simulink model "k1visetmxp"  (Simulink 8.6)
settings: Solver=ode45  StartTime=0.0  StopTime=10.0  RelTol=1e-3
libraries: cdsIPCx x51, cdsFilt x7, cdsCDI64 x6, cdsCDO64 x6, BIO_CD_DECODE_MASTER x6, BIO_CD_ENCODE_MASTER x5, CHK_DIO x5, dac x3, VIS_LIB x3, cdsBit2Word x2, cdsAdcx0 x1, cdsAdcx1 x1
settings Model: Creator=controls  LastModifiedBy=controls
settings DataIOCC: SignalLoggingSaveFormat=Dataset
settings OptimizationCC: ExpressionDepthLimit=128
settings DebuggingCC: UnderspecifiedInitializationDetection=Simplified  MergeDetectMultiDrivingBlocksExec=error  SolverPrmCheckMsg=none  FcnCallInpInsideContextMsg=EnableAllAsError  StateNameClashWarn=none
settings GRTTargetCC: CombineOutputUpdateFcns=on  GRTInterface=off

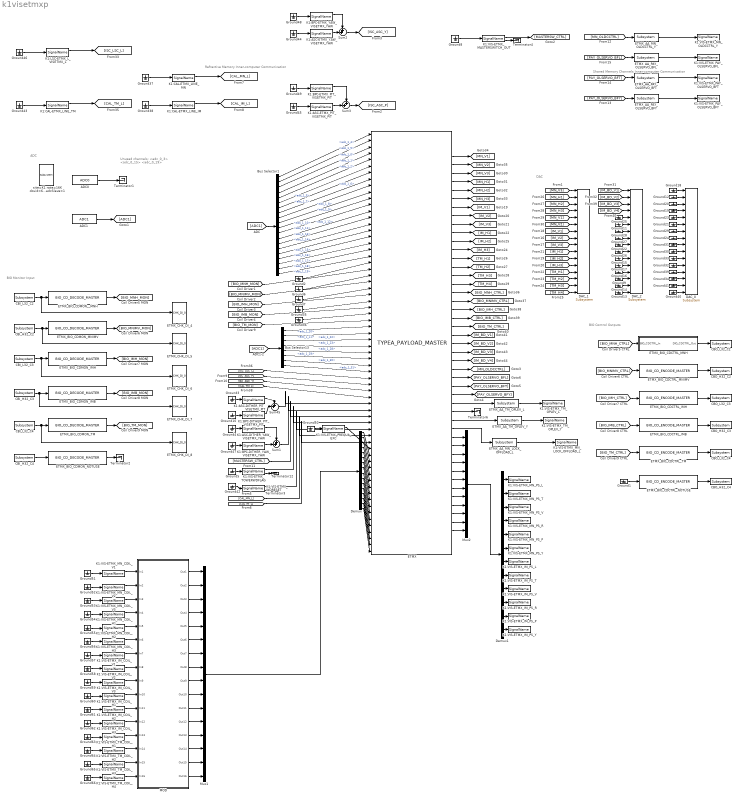
== system k1visetmxp ==
  note: BIO Monitor Input
  note: BIO Control Outputs
  note: DAC
  note: ADC
  note: Refrective Memory
      | Inner-computer Communication
  note: Unused channels:
      | <adc_0_3>
      | <adc_0_15>
      | <adc_0_19>
  note: Shared Memory Channels
      | Inner-computer Communication
  ADC0 : cdsAdcx0/ADC0  Tag=cdsAdc  Description=|
      | type-GSC_16AI64SSA
      | card_num=0
      settings: AttributesFormatString=%<Description>\n%<Tag>
  ADC1 : cdsAdcx1/ADC1  Tag=cdsAdc  Description=|
      | type-GSC_16AI64SSA
      | card_num=1
      settings: AttributesFormatString=%<Description>\n%<Tag>
  Bus Selector1 : BusSelector  OutputSignals=adc_1_4,adc_1_5,adc_1_0,adc_1_1,adc_1_2,adc_1_3,adc_1_6,adc_1_7,adc_1_8,adc_1_9,adc_1_10,adc_1_11,adc_1_12,adc_1_13,adc_1_14,adc_1_15,adc_1_16,adc_1_17,adc_1_18,adc_1_19
  Bus Selector13 : BusSelector  OutputSignals=adc_1_20,adc_1_21,adc_1_22,adc_1_23,adc_1_28,adc_1_29,adc_1_30,adc_1_31
  CBI_H32_C2 : cdsCDI64/Subsystem  Tag=cdsCDI64  Description=card_num=5
      settings: AttributesFormatString=%<Tag>\n%<Description>
  CBI_H32_C3 : cdsCDI64/Subsystem  Tag=cdsCDI64  Description=card_num=7
      settings: AttributesFormatString=%<Tag>\n%<Description>
  CBI_H32_C4 : cdsCDI64/Subsystem  Tag=cdsCDI64  Description=card_num=9
      settings: AttributesFormatString=%<Tag>\n%<Description>
  CBI_L32_C2 : cdsCDI64/Subsystem  Tag=cdsCDI64  Description=card_num=4
      settings: AttributesFormatString=%<Tag>\n%<Description>
  CBI_L32_C3 : cdsCDI64/Subsystem  Tag=cdsCDI64  Description=card_num=6
      settings: AttributesFormatString=%<Tag>\n%<Description>
  CBI_L32_C4 : cdsCDI64/Subsystem  Tag=cdsCDI64  Description=card_num=8
      settings: AttributesFormatString=%<Tag>\n%<Description>
  CBO_H32_C2 : cdsCDO64/Subsystem  Tag=cdsCDO64  Description=card_num=5
      settings: AttributesFormatString=%<Tag>\n%<Description>
  CBO_H32_C3 : cdsCDO64/Subsystem  Tag=cdsCDO64  Description=card_num=7
      settings: AttributesFormatString=%<Tag>\n%<Description>
  CBO_H32_C4 : cdsCDO64/Subsystem  Tag=cdsCDO64  Description=card_num=9
      settings: AttributesFormatString=%<Tag>\n%<Description>
  CBO_L32_C2 : cdsCDO64/Subsystem  Tag=cdsCDO64  Description=card_num=4
      settings: AttributesFormatString=%<Tag>\n%<Description>
  CBO_L32_C3 : cdsCDO64/Subsystem  Tag=cdsCDO64  Description=card_num=6
      settings: AttributesFormatString=%<Tag>\n%<Description>
  CBO_L32_C4 : cdsCDO64/Subsystem  Tag=cdsCDO64  Description=card_num=8
      settings: AttributesFormatString=%<Tag>\n%<Description>
  DAC_0 : dac/Subsystem  Description=|
      | type=GSC_16AO16,
      | card_num=0
      settings: AttributesFormatString=%<Description>
  DAC_1 : dac/Subsystem  Description=|
      | type=GSC_16AO16,
      | card_num=1
      settings: AttributesFormatString=%<Description>
  DAC_2 : dac/Subsystem  Description=|
      | type=GSC_16AO16,
      | card_num=2
      settings: AttributesFormatString=%<Description>
  Demux : Demux  Outputs=16
  Demux1 : Demux  Outputs=12
  ETMX : TYPEA_MASTER/TYPEA_PAYLOAD_MASTER
  ETMX_AA_MN_LOCK_OFFLOAD_L : cdsFilt/Subsystem  Tag=cdsFilt  Description=|
      | Purpose:                                                                                                                                                                                                                                  
      | Standard CDS IIR filter module.                                                                                                                                                                                                           
      |                                                                                                                                                                                                                                           
      | Operation:                                                                                                                                                                                                                                
      | Consists of 10 second order section IIR filters, plus a ramped gain stage. In FE code, also provides pre-defined test points and excitation channel inputs. The filter coefficients are defined in the LIGO system using the 'foton' tool.
      |                                                                                                                                                                                                                                           
      | Usage:                                                                                                                                                                                                                                    
      | Name the part with the desired filter module name.
      settings: AttributesFormatString=%<Tag>
  ETMX_AA_MN_OLDCCTRL_Y : cdsFilt/Subsystem  Tag=cdsFilt  Description=|
      | Purpose:                                                                                                                                                                                                                                  
      | Standard CDS IIR filter module.                                                                                                                                                                                                           
      |                                                                                                                                                                                                                                           
      | Operation:                                                                                                                                                                                                                                
      | Consists of 10 second order section IIR filters, plus a ramped gain stage. In FE code, also provides pre-defined test points and excitation channel inputs. The filter coefficients are defined in the LIGO system using the 'foton' tool.
      |                                                                                                                                                                                                                                           
      | Usage:                                                                                                                                                                                                                                    
      | Name the part with the desired filter module name.
      settings: AttributesFormatString=%<Tag>
  ETMX_AA_PAY_OLSERVO_BFL : cdsFilt/Subsystem  Tag=cdsFilt  Description=|
      | Purpose:                                                                                                                                                                                                                                  
      | Standard CDS IIR filter module.                                                                                                                                                                                                           
      |                                                                                                                                                                                                                                           
      | Operation:                                                                                                                                                                                                                                
      | Consists of 10 second order section IIR filters, plus a ramped gain stage. In FE code, also provides pre-defined test points and excitation channel inputs. The filter coefficients are defined in the LIGO system using the 'foton' tool.
      |                                                                                                                                                                                                                                           
      | Usage:                                                                                                                                                                                                                                    
      | Name the part with the desired filter module name.
      settings: AttributesFormatString=%<Tag>
  ETMX_AA_PAY_OLSERVO_BFT : cdsFilt/Subsystem  Tag=cdsFilt  Description=|
      | Purpose:                                                                                                                                                                                                                                  
      | Standard CDS IIR filter module.                                                                                                                                                                                                           
      |                                                                                                                                                                                                                                           
      | Operation:                                                                                                                                                                                                                                
      | Consists of 10 second order section IIR filters, plus a ramped gain stage. In FE code, also provides pre-defined test points and excitation channel inputs. The filter coefficients are defined in the LIGO system using the 'foton' tool.
      |                                                                                                                                                                                                                                           
      | Usage:                                                                                                                                                                                                                                    
      | Name the part with the desired filter module name.
      settings: AttributesFormatString=%<Tag>
  ETMX_AA_PAY_OLSERVO_BFY : cdsFilt/Subsystem  Tag=cdsFilt  Description=|
      | Purpose:                                                                                                                                                                                                                                  
      | Standard CDS IIR filter module.                                                                                                                                                                                                           
      |                                                                                                                                                                                                                                           
      | Operation:                                                                                                                                                                                                                                
      | Consists of 10 second order section IIR filters, plus a ramped gain stage. In FE code, also provides pre-defined test points and excitation channel inputs. The filter coefficients are defined in the LIGO system using the 'foton' tool.
      |                                                                                                                                                                                                                                           
      | Usage:                                                                                                                                                                                                                                    
      | Name the part with the desired filter module name.
      settings: AttributesFormatString=%<Tag>
  ETMX_AA_TM_OPLEV_L : cdsFilt/Subsystem  Tag=cdsFilt  Description=|
      | Purpose:                                                                                                                                                                                                                                  
      | Standard CDS IIR filter module.                                                                                                                                                                                                           
      |                                                                                                                                                                                                                                           
      | Operation:                                                                                                                                                                                                                                
      | Consists of 10 second order section IIR filters, plus a ramped gain stage. In FE code, also provides pre-defined test points and excitation channel inputs. The filter coefficients are defined in the LIGO system using the 'foton' tool.
      |                                                                                                                                                                                                                                           
      | Usage:                                                                                                                                                                                                                                    
      | Name the part with the desired filter module name.
      settings: AttributesFormatString=%<Tag>
  ETMX_AA_TM_OPLEV_Y : cdsFilt/Subsystem  Tag=cdsFilt  Description=|
      | Purpose:                                                                                                                                                                                                                                  
      | Standard CDS IIR filter module.                                                                                                                                                                                                           
      |                                                                                                                                                                                                                                           
      | Operation:                                                                                                                                                                                                                                
      | Consists of 10 second order section IIR filters, plus a ramped gain stage. In FE code, also provides pre-defined test points and excitation channel inputs. The filter coefficients are defined in the LIGO system using the 'foton' tool.
      |                                                                                                                                                                                                                                           
      | Usage:                                                                                                                                                                                                                                    
      | Name the part with the desired filter module name.
      settings: AttributesFormatString=%<Tag>
  ETMX_BIO_CDCTRL_IMB : BIO_CD_ENCODE_MASTER/BIO_CD_ENCODE_MASTER
  ETMX_BIO_CDCTRL_IMH : BIO_CD_ENCODE_MASTER/BIO_CD_ENCODE_MASTER
  ETMX_BIO_CDCTRL_MNH : Subsystem
  ETMX_BIO_CDCTRL_MNIMV : BIO_CD_ENCODE_MASTER/BIO_CD_ENCODE_MASTER
  ETMX_BIO_CDCTRL_NOTUSE : BIO_CD_ENCODE_MASTER/BIO_CD_ENCODE_MASTER
  ETMX_BIO_CDCTRL_TM : BIO_CD_ENCODE_MASTER/BIO_CD_ENCODE_MASTER
  ETMX_BIO_CDMON_IMB : BIO_CD_DECODE_MASTER/BIO_CD_DECODE_MASTER
  ETMX_BIO_CDMON_IMH : BIO_CD_DECODE_MASTER/BIO_CD_DECODE_MASTER
  ETMX_BIO_CDMON_MNIMV : BIO_CD_DECODE_MASTER/BIO_CD_DECODE_MASTER
  ETMX_BIO_CDMON_NOTUSE : BIO_CD_DECODE_MASTER/BIO_CD_DECODE_MASTER
  ETMX_BIO_CDMON_TM : BIO_CD_DECODE_MASTER/BIO_CD_DECODE_MASTER
  ETMX_BIO_CDMON__MNH : BIO_CD_DECODE_MASTER/BIO_CD_DECODE_MASTER
  ETMX_CHK_DI_{4..8} (5 alike) : CHK_DIO/CHK_DI_0
  Ground{1..66} (66 alike) : Ground
  K1:ASC-DITHER_PIT_VISETMX_PIT : cdsIPCx/SignalName  Tag=cdsIPCx_RFM  Description=card=0
      settings: AttributesFormatString=%<Description>\n%<Tag>
  K1:ASC-DITHER_YAW_VISETMX_YAW : cdsIPCx/SignalName  Tag=cdsIPCx_RFM  Description=card=0
      settings: AttributesFormatString=%<Description>\n%<Tag>
  K1:ASC-ETMX_PIT_VISETMX_PIT : cdsIPCx/SignalName  Tag=cdsIPCx_RFM  Description=card=0
      settings: AttributesFormatString=%<Description>\n%<Tag>
  K1:ASC-ETMX_YAW_VISETMX_YAW : cdsIPCx/SignalName  Tag=cdsIPCx_RFM  Description=card=0
      settings: AttributesFormatString=%<Description>\n%<Tag>
  K1:BPC-DITHER_PIT_VISETMX_PIT : cdsIPCx/SignalName  Tag=cdsIPCx_RFM  Description=card=0
      settings: AttributesFormatString=%<Description>\n%<Tag>
  K1:BPC-DITHER_YAW_VISETMX_YAW : cdsIPCx/SignalName  Tag=cdsIPCx_RFM  Description=card=0
      settings: AttributesFormatString=%<Description>\n%<Tag>
  K1:BPC-ETMX_PIT_VISETMX_PIT : cdsIPCx/SignalName  Tag=cdsIPCx_RFM  Description=card=0
      settings: AttributesFormatString=%<Description>\n%<Tag>
  K1:BPC-ETMX_YAW_VISETMX_YAW : cdsIPCx/SignalName  Tag=cdsIPCx_RFM  Description=card=0
      settings: AttributesFormatString=%<Description>\n%<Tag>
  K1:CAL-ETMX_LINE_IM : cdsIPCx/SignalName  Tag=cdsIPCx_RFM  Description=card=0
      settings: AttributesFormatString=%<Description>\n%<Tag>
  K1:CAL-ETMX_LINE_MN : cdsIPCx/SignalName  Tag=cdsIPCx_RFM  Description=card=0
      settings: AttributesFormatString=%<Description>\n%<Tag>
  K1:CAL-ETMX_LINE_TM : cdsIPCx/SignalName  Tag=cdsIPCx_RFM  Description=card=0
      settings: AttributesFormatString=%<Description>\n%<Tag>
  K1:LSC-ETMX_L_VISETMX_L : cdsIPCx/SignalName  Tag=cdsIPCx_RFM  Description=card=0
      settings: AttributesFormatString=%<Description>\n%<Tag>
  K1:VIS-ETMX_MASTERSWITCH_OUT : cdsIPCx/SignalName  Tag=cdsIPCx_SHMEM  Description=Inter-Process Communication via Shared memory.
      settings: AttributesFormatString=%<Tag>
  K1:VIS-ETMX_MN_LOCK_OFFLOAD_L : cdsIPCx/SignalName  Tag=cdsIPCx_SHMEM  Description=Inter-Process Communication via Shared memory.
      settings: AttributesFormatString=%<Tag>
  K1:VIS-ETMX_MN_OLDCCTRL_Y : cdsIPCx/SignalName  Tag=cdsIPCx_SHMEM  Description=Inter-Process Communication via Shared memory.
      settings: AttributesFormatString=%<Tag>
  K1:VIS-ETMX_PAY_OLSERVO_BFL : cdsIPCx/SignalName  Tag=cdsIPCx_SHMEM  Description=Inter-Process Communication via Shared memory.
      settings: AttributesFormatString=%<Tag>
  K1:VIS-ETMX_PAY_OLSERVO_BFT : cdsIPCx/SignalName  Tag=cdsIPCx_SHMEM  Description=Inter-Process Communication via Shared memory.
      settings: AttributesFormatString=%<Tag>
  K1:VIS-ETMX_PAY_OLSERVO_BFY : cdsIPCx/SignalName  Tag=cdsIPCx_SHMEM  Description=Inter-Process Communication via Shared memory.
      settings: AttributesFormatString=%<Tag>
  K1:VIS-ETMX_TM_OPLEV_L : cdsIPCx/SignalName  Tag=cdsIPCx_SHMEM  Description=Inter-Process Communication via Shared memory.
      settings: AttributesFormatString=%<Tag>
  K1:VIS-ETMX_TM_OPLEV_Y : cdsIPCx/SignalName  Tag=cdsIPCx_SHMEM  Description=Inter-Process Communication via Shared memory.
      settings: AttributesFormatString=%<Tag>
  K1:VIS-ETMX_TOWERWDFLAG : cdsIPCx/SignalName  Tag=cdsIPCx_SHMEM  Description=Inter-Process Communication via Shared memory.
      settings: AttributesFormatString=%<Tag>
  K1:VIS-ETMX_WDRESET : cdsIPCx/SignalName  Tag=cdsIPCx_SHMEM  Description=Inter-Process Communication via Shared memory.
      settings: AttributesFormatString=%<Tag>
  K1:VIS-ETMX_IM_COIL_H1 : cdsIPCx/SignalName  Tag=cdsIPCx_SHMEM  Description=Inter-Process Communication via Shared memory.
      settings: AttributesFormatString=%<Tag>
  K1:VIS-ETMX_IM_COIL_H2 : cdsIPCx/SignalName  Tag=cdsIPCx_SHMEM  Description=Inter-Process Communication via Shared memory.
      settings: AttributesFormatString=%<Tag>
  K1:VIS-ETMX_IM_COIL_H3 : cdsIPCx/SignalName  Tag=cdsIPCx_SHMEM  Description=Inter-Process Communication via Shared memory.
      settings: AttributesFormatString=%<Tag>
  K1:VIS-ETMX_IM_COIL_V1 : cdsIPCx/SignalName  Tag=cdsIPCx_SHMEM  Description=Inter-Process Communication via Shared memory.
      settings: AttributesFormatString=%<Tag>
  K1:VIS-ETMX_IM_COIL_V2 : cdsIPCx/SignalName  Tag=cdsIPCx_SHMEM  Description=Inter-Process Communication via Shared memory.
      settings: AttributesFormatString=%<Tag>
  K1:VIS-ETMX_IM_COIL_V3 : cdsIPCx/SignalName  Tag=cdsIPCx_SHMEM  Description=Inter-Process Communication via Shared memory.
      settings: AttributesFormatString=%<Tag>
  K1:VIS-ETMX_IM_PS_L : cdsIPCx/SignalName  Tag=cdsIPCx_SHMEM  Description=Inter-Process Communication via Shared memory.
      settings: AttributesFormatString=%<Tag>
  K1:VIS-ETMX_IM_PS_P : cdsIPCx/SignalName  Tag=cdsIPCx_SHMEM  Description=Inter-Process Communication via Shared memory.
      settings: AttributesFormatString=%<Tag>
  K1:VIS-ETMX_IM_PS_R : cdsIPCx/SignalName  Tag=cdsIPCx_SHMEM  Description=Inter-Process Communication via Shared memory.
      settings: AttributesFormatString=%<Tag>
  K1:VIS-ETMX_IM_PS_T : cdsIPCx/SignalName  Tag=cdsIPCx_SHMEM  Description=Inter-Process Communication via Shared memory.
      settings: AttributesFormatString=%<Tag>
  K1:VIS-ETMX_IM_PS_V : cdsIPCx/SignalName  Tag=cdsIPCx_SHMEM  Description=Inter-Process Communication via Shared memory.
      settings: AttributesFormatString=%<Tag>
  K1:VIS-ETMX_IM_PS_Y : cdsIPCx/SignalName  Tag=cdsIPCx_SHMEM  Description=Inter-Process Communication via Shared memory.
      settings: AttributesFormatString=%<Tag>
  K1:VIS-ETMX_MN_COIL_H1 : cdsIPCx/SignalName  Tag=cdsIPCx_SHMEM  Description=Inter-Process Communication via Shared memory.
      settings: AttributesFormatString=%<Tag>
  K1:VIS-ETMX_MN_COIL_H2 : cdsIPCx/SignalName  Tag=cdsIPCx_SHMEM  Description=Inter-Process Communication via Shared memory.
      settings: AttributesFormatString=%<Tag>
  K1:VIS-ETMX_MN_COIL_H3 : cdsIPCx/SignalName  Tag=cdsIPCx_SHMEM  Description=Inter-Process Communication via Shared memory.
      settings: AttributesFormatString=%<Tag>
  K1:VIS-ETMX_MN_COIL_V1 : cdsIPCx/SignalName  Tag=cdsIPCx_SHMEM  Description=Inter-Process Communication via Shared memory.
      settings: AttributesFormatString=%<Tag>
  K1:VIS-ETMX_MN_COIL_V2 : cdsIPCx/SignalName  Tag=cdsIPCx_SHMEM  Description=Inter-Process Communication via Shared memory.
      settings: AttributesFormatString=%<Tag>
  K1:VIS-ETMX_MN_COIL_V3 : cdsIPCx/SignalName  Tag=cdsIPCx_SHMEM  Description=Inter-Process Communication via Shared memory.
      settings: AttributesFormatString=%<Tag>
  K1:VIS-ETMX_MN_PS_L : cdsIPCx/SignalName  Tag=cdsIPCx_SHMEM  Description=Inter-Process Communication via Shared memory.
      settings: AttributesFormatString=%<Tag>
  K1:VIS-ETMX_MN_PS_P : cdsIPCx/SignalName  Tag=cdsIPCx_SHMEM  Description=Inter-Process Communication via Shared memory.
      settings: AttributesFormatString=%<Tag>
  K1:VIS-ETMX_MN_PS_R : cdsIPCx/SignalName  Tag=cdsIPCx_SHMEM  Description=Inter-Process Communication via Shared memory.
      settings: AttributesFormatString=%<Tag>
  K1:VIS-ETMX_MN_PS_T : cdsIPCx/SignalName  Tag=cdsIPCx_SHMEM  Description=Inter-Process Communication via Shared memory.
      settings: AttributesFormatString=%<Tag>
  K1:VIS-ETMX_MN_PS_V : cdsIPCx/SignalName  Tag=cdsIPCx_SHMEM  Description=Inter-Process Communication via Shared memory.
      settings: AttributesFormatString=%<Tag>
  K1:VIS-ETMX_MN_PS_Y : cdsIPCx/SignalName  Tag=cdsIPCx_SHMEM  Description=Inter-Process Communication via Shared memory.
      settings: AttributesFormatString=%<Tag>
  K1:VIS-ETMX_PREQUA_EXC : cdsIPCx/SignalName  Tag=cdsIPCx_SHMEM  Description=Inter-Process Communication via Shared memory.
      settings: AttributesFormatString=%<Tag>
  K1:VIS-ETMX_TM_COIL_H{1..4} (4 alike) : cdsIPCx/SignalName  Tag=cdsIPCx_SHMEM  Description=Inter-Process Communication via Shared memory.
      settings: AttributesFormatString=%<Tag>
  MOD : Subsystem  Tag=top_names
  Mux1 : Mux  Inputs=16
  Mux2 : Mux  Inputs=12
  Sum{1..3,45} (4 alike) : Sum  Inputs=++|
  Terminator{1..4,6,12} (6 alike) : Terminator
  site=K1 rate=16K dcuid=69 host=k1ex1 specific_cpu=3 adcSlave=1 : cdsParameters/Subsystem  Tag=cdsParameters  Description=|
      | Purpose:                                                                                                                                                                                                                                
      | Provide system parameters to the FE code generator to properly configure the generated EPICS names, rep rate of the FE controller, and the Data Acquisition node ID for proper storage of data from this FE controller.                 
      |                                                                                                                                                                                                                                         
      | Useage:                                                                                                                                                                                                                                 
      | The part NAME field is used to identify the FE parameters. It must be of the form:                                                                                                                                                      
      | site=                                                                                                                                                                                                                                   
      | rate=                                                                                                                                                                                                                                   
      | dcuid=                                                                                                                                                                                                                                  
      |                                                                                                                                                                                                                                         
      | Where:                                                                                                                                                                                                                                  
      | site= argument may be H1, H2, L1, M1, G1, either as a single argument or multiple, for example site=H1,H2. These are the only names allowed. These will become the first two characters of all EPICS and signal names (for example G1:).
      |                                                                                                                                                                                                                                         
      | rate= may be 2K, 16K, 32K, or 64K                                                                                                                                                                                                       
      |                                                                                                                                                                                                                                         
      | dcuid= is site specific ie it must be unique at each site.
      settings: AttributesFormatString=%<Tag>
  wires:
  ADC1/1 -> [ADC1]
  ETMX/1 -> [MN_V1]
  ETMX/2 -> [MN_V2]
  ETMX/3 -> [MN_V3]
  ETMX/4 -> [MN_H1]
  ETMX/6 -> [MN_H3]
  ETMX/7 -> [IM_V1]
  ETMX/8 -> [IM_V2]
  ETMX/9 -> [IM_V3]
  ETMX/11 -> [IM_H2]
  ETMX/12 -> [IM_H3]
  ETMX/13 -> [TM_H1]
  ETMX/14 -> [TM_H2]
  ETMX/16 -> [TM_H4]
  ETMX/17 -> [BIO_MNH_CTRL]
  ETMX/19 -> [BIO_IMH_CTRL]
  ETMX/18 -> [BIO_MNIMV_CTRL]
  ETMX/20 -> [BIO_IMB_CTRL]
  ETMX/21 -> [BIO_TM_CTRL]
  [ADC1] -> Bus Selector13/1
  [MN_V3] -> DAC_1/1
  [MN_H1] -> DAC_1/2
  [MN_H2] -> DAC_1/3
  [MN_H3] -> DAC_1/4
  [MN_V1] -> DAC_1/5
  [MN_V2] -> DAC_1/6
  [IM_V1] -> DAC_1/7
  [IM_V2] -> DAC_1/8
  [IM_V3] -> DAC_1/9
  [IM_H1] -> DAC_1/10
  [TM_H1] -> DAC_1/13
  [TM_H4] -> DAC_1/16
  [TM_H3] -> DAC_1/15
  [TM_H2] -> DAC_1/14
  [IM_H2] -> DAC_1/11
  [IM_H3] -> DAC_1/12
  [BIO_MNH_CTRL] -> ETMX_BIO_CDCTRL_MNH/1(BIO_CDCTRL_In)
  ETMX_BIO_CDCTRL_MNH/1(DIO_CDCTRL_Out) -> CBO_L32_C2/1
  [BIO_MNIMV_CTRL] -> ETMX_BIO_CDCTRL_MNIMV/1
  ETMX_BIO_CDCTRL_MNIMV/1 -> CBO_H32_C2/1
  [BIO_IMH_CTRL] -> ETMX_BIO_CDCTRL_IMH/1
  ETMX_BIO_CDCTRL_IMH/1 -> CBO_L32_C3/1
  [BIO_IMB_CTRL] -> ETMX_BIO_CDCTRL_IMB/1
  ETMX_BIO_CDCTRL_IMB/1 -> CBO_H32_C3/1
  [BIO_TM_CTRL] -> ETMX_BIO_CDCTRL_TM/1
  ETMX_BIO_CDCTRL_TM/1 -> CBO_L32_C4/1
  Ground1/1 -> ETMX_BIO_CDCTRL_NOTUSE/1
  ETMX_BIO_CDCTRL_NOTUSE/1 -> CBO_H32_C4/1
  CBI_L32_C2/1 -> ETMX_CHK_DI_4/1, ETMX_BIO_CDMON__MNH/1
  ETMX_BIO_CDMON__MNH/1 -> [BIO_MNH_MON]
  CBI_H32_C2/1 -> ETMX_CHK_DI_5/1, ETMX_BIO_CDMON_MNIMV/1
  ETMX_BIO_CDMON_MNIMV/1 -> [BIO_MNIMV_MON]
  CBI_L32_C3/1 -> ETMX_CHK_DI_6/1, ETMX_BIO_CDMON_IMH/1
  ETMX_BIO_CDMON_IMH/1 -> [BIO_IMH_MON]
  ETMX_BIO_CDMON_IMB/1 -> [BIO_IMB_MON]
  CBI_L32_C4/1 -> ETMX_CHK_DI_8/1, ETMX_BIO_CDMON_TM/1
  ETMX_BIO_CDMON_TM/1 -> [BIO_TM_MON]
  CBI_H32_C4/1 -> ETMX_BIO_CDMON_NOTUSE/1
  ETMX_BIO_CDMON_NOTUSE/1 -> Terminator2/1
  [IM_BD_V1] -> DAC_2/1
  [IM_BD_V2] -> DAC_2/2
  [IM_BD_V3] -> DAC_2/3
  [IM_BD_V4] -> DAC_2/4
  Ground25/1 -> DAC_2/5
  Ground11/1 -> DAC_2/6
  Ground28/1 -> DAC_2/7
  Ground27/1 -> DAC_2/8
  Ground22/1 -> DAC_2/9
  Ground26/1 -> DAC_2/10
  Ground15/1 -> DAC_2/11
  Ground17/1 -> DAC_2/12
  Ground16/1 -> DAC_2/13
  Ground9/1 -> DAC_2/14
  Ground14/1 -> DAC_2/15
  Ground13/1 -> DAC_2/16
  ETMX/22 -> [IM_BD_V1]
  ETMX/23 -> [IM_BD_V2]
  ETMX/24 -> [IM_BD_V3]
  ETMX/25 -> [IM_BD_V4]
  CBI_H32_C3/1 -> ETMX_CHK_DI_7/1, ETMX_BIO_CDMON_IMB/1
  ETMX/5 -> [MN_H2]
  ETMX/10 -> [IM_H1]
  ETMX/15 -> [TM_H3]
  [ADC1] -> Bus Selector1/1
  K1:VIS-ETMX_TOWERWDFLAG/2 -> Terminator12/1
  Ground5/1 -> K1:VIS-ETMX_TOWERWDFLAG/1
  ADC0/1 -> Terminator1/1
  Ground18/1 -> DAC_0/1
  Ground12/1 -> DAC_0/2
  Ground19/1 -> DAC_0/4
  Ground20/1 -> DAC_0/3
  Ground29/1 -> DAC_0/7
  Ground23/1 -> DAC_0/5
  Ground21/1 -> DAC_0/6
  Ground24/1 -> DAC_0/8
  Ground31/1 -> DAC_0/9
  Ground30/1 -> DAC_0/10
  Ground33/1 -> DAC_0/11
  Ground32/1 -> DAC_0/12
  Ground39/1 -> DAC_0/13
  Ground34/1 -> DAC_0/14
  Ground41/1 -> DAC_0/15
  Ground40/1 -> DAC_0/16
  K1:VIS-ETMX_WDRESET/2 -> Terminator3/1
  Ground42/1 -> K1:VIS-ETMX_WDRESET/1
  Ground46/1 -> K1:LSC-ETMX_L_VISETMX_L/1
  K1:LSC-ETMX_L_VISETMX_L/1 -> [ISC_LSC_L]
  K1:CAL-ETMX_LINE_TM/1 -> [CAL_TM_L]
  Ground43/1 -> K1:CAL-ETMX_LINE_TM/1
  K1:CAL-ETMX_LINE_MN/1 -> [CAL_MN_L]
  Ground37/1 -> K1:CAL-ETMX_LINE_MN/1
  K1:CAL-ETMX_LINE_IM/1 -> [CAL_IM_L]
  Ground38/1 -> K1:CAL-ETMX_LINE_IM/1
  Ground44/1 -> K1:ASC-ETMX_YAW_VISETMX_YAW/1
  Ground45/1 -> K1:ASC-ETMX_PIT_VISETMX_PIT/1
  K1:ASC-ETMX_YAW_VISETMX_YAW/1 -> Sum2/2
  K1:ASC-ETMX_PIT_VISETMX_PIT/1 -> Sum3/2
  Ground3/1 -> K1:ASC-DITHER_PIT_VISETMX_PIT/1
  Ground4/1 -> K1:ASC-DITHER_YAW_VISETMX_YAW/1
  ETMX_AA_MN_OLDCCTRL_Y/1 -> K1:VIS-ETMX_MN_OLDCCTRL_Y/1
  ETMX_AA_PAY_OLSERVO_BFY/1 -> K1:VIS-ETMX_PAY_OLSERVO_BFY/1
  ETMX_AA_PAY_OLSERVO_BFT/1 -> K1:VIS-ETMX_PAY_OLSERVO_BFT/1
  ETMX_AA_PAY_OLSERVO_BFL/1 -> K1:VIS-ETMX_PAY_OLSERVO_BFL/1
  [PAY_OLSERVO_BFY] -> ETMX_AA_PAY_OLSERVO_BFY/1
  [PAY_OLSERVO_BFT] -> ETMX_AA_PAY_OLSERVO_BFT/1
  [PAY_OLSERVO_BFL] -> ETMX_AA_PAY_OLSERVO_BFL/1
  [MN_OLDCCTRL] -> ETMX_AA_MN_OLDCCTRL_Y/1
  ETMX_AA_TM_OPLEV_L/1 -> K1:VIS-ETMX_TM_OPLEV_L/1
  ETMX_AA_TM_OPLEV_Y/1 -> K1:VIS-ETMX_TM_OPLEV_Y/1
  Bus Selector13/1 -> ETMX/31  "<adc_1_20>"
  Bus Selector13/2 -> ETMX/32  "<adc_1_21>"
  Bus Selector13/3 -> ETMX/33  "<adc_1_22>"
  Bus Selector1/19 -> ETMX/19  "<adc_1_18>"
  Bus Selector1/20 -> ETMX/20  "<adc_1_19>"
  Bus Selector1/5 -> ETMX/5  "<adc_1_2>"
  Bus Selector1/16 -> ETMX/16  "<adc_1_15>"
  Bus Selector1/17 -> ETMX/17  "<adc_1_16>"
  Bus Selector1/18 -> ETMX/18  "<adc_1_17>"
  Bus Selector13/4 -> ETMX/34  "<adc_1_23>"
  Bus Selector13/5 -> ETMX/35  "<adc_1_28>"
  Bus Selector13/6 -> ETMX/36  "<adc_1_29>"
  Bus Selector13/7 -> ETMX/37  "<adc_1_30>"
  Bus Selector1/3 -> ETMX/3  "<adc_1_0>"
  Bus Selector1/10 -> ETMX/10  "<adc_1_9>"
  Bus Selector1/11 -> ETMX/11  "<adc_1_10>"
  Bus Selector1/8 -> ETMX/8  "<adc_1_7>"
  Bus Selector1/9 -> ETMX/9  "<adc_1_8>"
  Bus Selector1/14 -> ETMX/14  "<adc_1_13>"
  Bus Selector1/15 -> ETMX/15  "<adc_1_14>"
  Bus Selector1/12 -> ETMX/12  "<adc_1_11>"
  Bus Selector1/13 -> ETMX/13  "<adc_1_12>"
  Bus Selector1/4 -> ETMX/4  "<adc_1_1>"
  Bus Selector1/2 -> ETMX/2  "<adc_1_5>"
  Bus Selector1/1 -> ETMX/1  "<adc_1_4>"
  Bus Selector13/8 -> ETMX/38  "<adc_1_31>"
  Bus Selector1/6 -> ETMX/6  "<adc_1_3>"
  Bus Selector1/7 -> ETMX/7  "<adc_1_6>"
  Ground35/1 -> ETMX/27
  Ground36/1 -> ETMX/29
  Ground2/1 -> ETMX/21
  Ground6/1 -> ETMX/23
  Ground7/1 -> ETMX/25
  [ISC_ASC_Y] -> ETMX/41
  [ISC_ASC_P] -> ETMX/40
  [ISC_LSC_L] -> ETMX/39
  [BIO_IMB_MON] -> ETMX/28
  [BIO_TM_MON] -> ETMX/30
  [BIO_MNH_MON] -> ETMX/22
  [BIO_MNIMV_MON] -> ETMX/24
  [BIO_IMH_MON] -> ETMX/26
  [CAL_IM_L] -> ETMX/49
  ETMX/26 -> [MN_OLDCCTRL]
  ETMX/27 -> [PAY_OLSERVO_BFL]
  ETMX/28 -> [PAY_OLSERVO_BFT]
  ETMX/29 -> [PAY_OLSERVO_BFY]
  ETMX/30 -> ETMX_AA_TM_OPLEV_L/1
  ETMX/31 -> Terminator6/1
  ETMX/32 -> ETMX_AA_TM_OPLEV_Y/1
  K1:VIS-ETMX_MASTERSWITCH_OUT/1 -> [MASTERSW_CTRL]
  Ground8/1 -> K1:VIS-ETMX_MASTERSWITCH_OUT/1
  K1:VIS-ETMX_MASTERSWITCH_OUT/2 -> Terminator4/1
  ETMX_AA_MN_LOCK_OFFLOAD_L/1 -> K1:VIS-ETMX_MN_LOCK_OFFLOAD_L/1
  ETMX/33 -> ETMX_AA_MN_LOCK_OFFLOAD_L/1
  [CAL_TM_L] -> ETMX/42
  K1:ASC-DITHER_PIT_VISETMX_PIT/1 -> Sum45/1
  K1:ASC-DITHER_YAW_VISETMX_YAW/1 -> Sum1/1
  [MASTERSW_CTRL] -> ETMX/45
  K1:VIS-ETMX_TOWERWDFLAG/1 -> ETMX/46
  K1:VIS-ETMX_WDRESET/1 -> ETMX/47
  [CAL_MN_L] -> ETMX/48
  Ground10/1 -> K1:BPC-DITHER_PIT_VISETMX_PIT/1
  Ground47/1 -> K1:BPC-DITHER_YAW_VISETMX_YAW/1
  K1:BPC-DITHER_PIT_VISETMX_PIT/1 -> Sum45/2
  Sum45/1 -> ETMX/43
  K1:BPC-DITHER_YAW_VISETMX_YAW/1 -> Sum1/2
  Sum1/1 -> ETMX/44
  Ground48/1 -> K1:BPC-ETMX_YAW_VISETMX_YAW/1
  Ground49/1 -> K1:BPC-ETMX_PIT_VISETMX_PIT/1
  Sum2/1 -> [ISC_ASC_Y]
  K1:BPC-ETMX_YAW_VISETMX_YAW/1 -> Sum2/1
  Sum3/1 -> [ISC_ASC_P]
  K1:BPC-ETMX_PIT_VISETMX_PIT/1 -> Sum3/1
  Mux1/1 -> Demux/1
  Ground51/1 -> K1:VIS-ETMX_MN_COIL_V1/1
  Ground66/1 -> K1:VIS-ETMX_TM_COIL_H4/1
  Ground52/1 -> K1:VIS-ETMX_MN_COIL_V2/1
  Ground53/1 -> K1:VIS-ETMX_MN_COIL_V3/1
  Ground54/1 -> K1:VIS-ETMX_MN_COIL_H1/1
  Ground55/1 -> K1:VIS-ETMX_MN_COIL_H2/1
  Ground56/1 -> K1:VIS-ETMX_MN_COIL_H3/1
  Ground57/1 -> K1:VIS-ETMX_IM_COIL_V1/1
  Ground58/1 -> K1:VIS-ETMX_IM_COIL_V2/1
  Ground59/1 -> K1:VIS-ETMX_IM_COIL_V3/1
  Ground60/1 -> K1:VIS-ETMX_IM_COIL_H1/1
  Ground61/1 -> K1:VIS-ETMX_IM_COIL_H2/1
  Ground62/1 -> K1:VIS-ETMX_IM_COIL_H3/1
  Ground63/1 -> K1:VIS-ETMX_TM_COIL_H1/1
  Ground64/1 -> K1:VIS-ETMX_TM_COIL_H2/1
  Ground65/1 -> K1:VIS-ETMX_TM_COIL_H3/1
  MOD/1(Out1) -> Mux1/1
  MOD/2(Out2) -> Mux1/2
  MOD/3(Out3) -> Mux1/3
  MOD/4(Out4) -> Mux1/4
  MOD/5(Out5) -> Mux1/5
  MOD/6(Out6) -> Mux1/6
  MOD/7(Out7) -> Mux1/7
  MOD/8(Out8) -> Mux1/8
  MOD/9(Out9) -> Mux1/9
  MOD/10(Out10) -> Mux1/10
  MOD/11(Out11) -> Mux1/11
  MOD/12(Out12) -> Mux1/12
  MOD/13(Out13) -> Mux1/13
  MOD/14(Out14) -> Mux1/14
  MOD/15(Out15) -> Mux1/15
  MOD/16(Out16) -> Mux1/16
  K1:VIS-ETMX_MN_COIL_V1/1 -> MOD/1(In1)
  K1:VIS-ETMX_MN_COIL_V2/1 -> MOD/2(In2)
  K1:VIS-ETMX_MN_COIL_V3/1 -> MOD/3(In3)
  K1:VIS-ETMX_MN_COIL_H1/1 -> MOD/4(In4)
  K1:VIS-ETMX_MN_COIL_H2/1 -> MOD/5(In5)
  K1:VIS-ETMX_MN_COIL_H3/1 -> MOD/6(In6)
  K1:VIS-ETMX_IM_COIL_V1/1 -> MOD/7(In7)
  K1:VIS-ETMX_IM_COIL_V2/1 -> MOD/8(In8)
  K1:VIS-ETMX_IM_COIL_V3/1 -> MOD/9(In9)
  K1:VIS-ETMX_IM_COIL_H1/1 -> MOD/10(In10)
  K1:VIS-ETMX_IM_COIL_H2/1 -> MOD/11(In11)
  K1:VIS-ETMX_IM_COIL_H3/1 -> MOD/12(In12)
  K1:VIS-ETMX_TM_COIL_H1/1 -> MOD/13(In13)
  K1:VIS-ETMX_TM_COIL_H2/1 -> MOD/14(In14)
  K1:VIS-ETMX_TM_COIL_H3/1 -> MOD/15(In15)
  K1:VIS-ETMX_TM_COIL_H4/1 -> MOD/16(In16)
  Demux/1 -> ETMX/51
  Demux/2 -> ETMX/52
  Demux/3 -> ETMX/53
  Demux/4 -> ETMX/54
  Demux/5 -> ETMX/55
  Demux/6 -> ETMX/56
  Demux/7 -> ETMX/57
  Demux/8 -> ETMX/58
  Demux/9 -> ETMX/59
  Demux/10 -> ETMX/60
  Demux/11 -> ETMX/61
  Demux/12 -> ETMX/62
  Demux/13 -> ETMX/63
  Demux/14 -> ETMX/64
  Demux/15 -> ETMX/65
  Demux/16 -> ETMX/66
  Ground50/1 -> K1:VIS-ETMX_PREQUA_EXC/1
  K1:VIS-ETMX_PREQUA_EXC/1 -> ETMX/50
  Demux1/1 -> K1:VIS-ETMX_MN_PS_L/1
  Demux1/2 -> K1:VIS-ETMX_MN_PS_T/1
  Demux1/3 -> K1:VIS-ETMX_MN_PS_V/1
  Demux1/4 -> K1:VIS-ETMX_MN_PS_R/1
  Demux1/5 -> K1:VIS-ETMX_MN_PS_P/1
  Demux1/6 -> K1:VIS-ETMX_MN_PS_Y/1
  Demux1/7 -> K1:VIS-ETMX_IM_PS_L/1
  Demux1/8 -> K1:VIS-ETMX_IM_PS_T/1
  Demux1/9 -> K1:VIS-ETMX_IM_PS_V/1
  Demux1/10 -> K1:VIS-ETMX_IM_PS_R/1
  Demux1/11 -> K1:VIS-ETMX_IM_PS_P/1
  Demux1/12 -> K1:VIS-ETMX_IM_PS_Y/1
  Mux2/1 -> Demux1/1
  ETMX/34 -> Mux2/1
  ETMX/35 -> Mux2/2
  ETMX/36 -> Mux2/3
  ETMX/37 -> Mux2/4
  ETMX/38 -> Mux2/5
  ETMX/39 -> Mux2/6
  ETMX/40 -> Mux2/7
  ETMX/41 -> Mux2/8
  ETMX/42 -> Mux2/9
  ETMX/43 -> Mux2/10
  ETMX/44 -> Mux2/11
  ETMX/45 -> Mux2/12

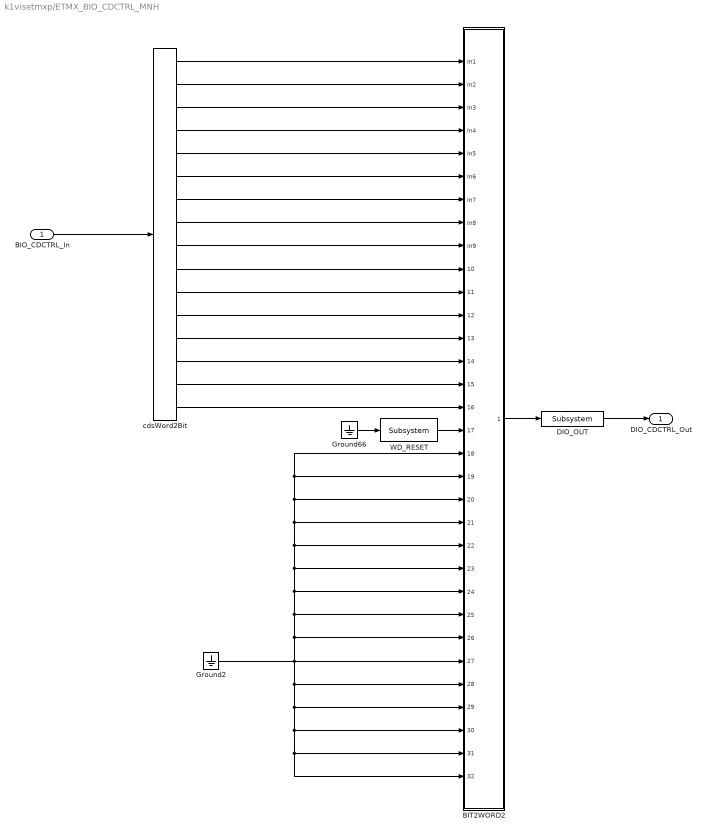
== system k1visetmxp/ETMX_BIO_CDCTRL_MNH ==
  BIO_CDCTRL_In : Inport
  BIT2WORD2 : Subsystem
  DIO_OUT : cdsEpicsOut/Subsystem  Tag=cdsEpicsOutput  Description=|
      | Purpose:                                          
      | Output a FE signal to an EPICS channel.           
      |                                                   
      | Operation:                                        
      | Takes input value and passes it to EPICS record.  
      |                                                   
      | Usage:                                            
      | Name the part with the desired EPICS rrecord name.
      settings: AttributesFormatString=%<Tag>
  Ground2 : Ground
  Ground66 : Ground
  WD_RESET : cdsEpicsBinIn/Subsystem  Tag=cdsEpicsBinIn  Description=|
      | Purpose:                                                                            
      | Create an EPICS binary (0 or 1) input channel to the FE realtime controls.          
      |                                                                                     
      | Operation:                                                                          
      | Outputs value from an EPICS ai record. Value is binary input (bi Epics record type).
      |                                                                                     
      | Usage:                                                                              
      | Name the part with the desired EPICS channel name.
      settings: AttributesFormatString=%<Tag>
  cdsWord2Bit : cdsWord2Bit/cdsWord2Bit  Tag=cdsWord2Bit  Description=Generate 16 0/1 outputs from single 16-bit integer input
      settings: AttributesFormatString=cdsWord2Bit
  DIO_CDCTRL_Out : Outport
  wires:
  BIT2WORD2/1(Out1) -> DIO_OUT/1
  DIO_OUT/1 -> DIO_CDCTRL_Out/1
  BIO_CDCTRL_In/1 -> cdsWord2Bit/1
  cdsWord2Bit/1 -> BIT2WORD2/1(In1)
  cdsWord2Bit/2 -> BIT2WORD2/2(In2)
  cdsWord2Bit/3 -> BIT2WORD2/3(In3)
  cdsWord2Bit/4 -> BIT2WORD2/4(In4)
  cdsWord2Bit/5 -> BIT2WORD2/5(In5)
  cdsWord2Bit/6 -> BIT2WORD2/6(In6)
  cdsWord2Bit/7 -> BIT2WORD2/7(In7)
  cdsWord2Bit/8 -> BIT2WORD2/8(In8)
  cdsWord2Bit/9 -> BIT2WORD2/9(In9)
  cdsWord2Bit/10 -> BIT2WORD2/10(In10)
  cdsWord2Bit/11 -> BIT2WORD2/11(In11)
  cdsWord2Bit/12 -> BIT2WORD2/12(In12)
  cdsWord2Bit/13 -> BIT2WORD2/13(In13)
  cdsWord2Bit/14 -> BIT2WORD2/14(In14)
  cdsWord2Bit/15 -> BIT2WORD2/15(In15)
  cdsWord2Bit/16 -> BIT2WORD2/16(In16)
  WD_RESET/1 -> BIT2WORD2/17(In17)
  Ground66/1 -> WD_RESET/1
  Ground2/1 -> BIT2WORD2/27(In27), BIT2WORD2/28(In28), BIT2WORD2/29(In29), BIT2WORD2/30(In30), BIT2WORD2/31(In31), BIT2WORD2/32(In32), BIT2WORD2/26(In26), BIT2WORD2/25(In25), BIT2WORD2/24(In24), BIT2WORD2/23(In23), BIT2WORD2/22(In22), BIT2WORD2/21(In21), BIT2WORD2/20(In20), BIT2WORD2/18(In18), BIT2WORD2/19(In19)

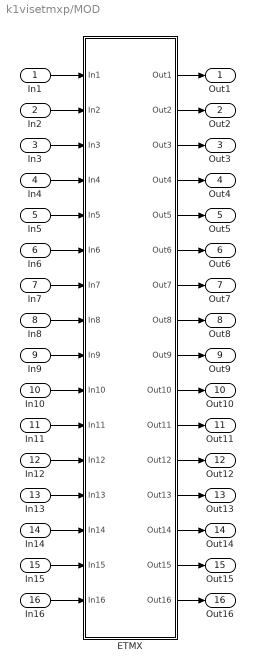
== system k1visetmxp/MOD ==
  In1 : Inport
  In2 : Inport  Port=2
  In3 : Inport  Port=3
  In4 : Inport  Port=4
  In5 : Inport  Port=5
  In6 : Inport  Port=6
  In7 : Inport  Port=7
  In8 : Inport  Port=8
  In9 : Inport  Port=9
  In10 : Inport  Port=10
  In11 : Inport  Port=11
  In12 : Inport  Port=12
  In13 : Inport  Port=13
  In14 : Inport  Port=14
  In15 : Inport  Port=15
  In16 : Inport  Port=16
  ETMX : Subsystem
  Out1 : Outport
  Out2 : Outport  Port=2
  Out3 : Outport  Port=3
  Out4 : Outport  Port=4
  Out5 : Outport  Port=5
  Out6 : Outport  Port=6
  Out7 : Outport  Port=7
  Out8 : Outport  Port=8
  Out9 : Outport  Port=9
  Out10 : Outport  Port=10
  Out11 : Outport  Port=11
  Out12 : Outport  Port=12
  Out13 : Outport  Port=13
  Out14 : Outport  Port=14
  Out15 : Outport  Port=15
  Out16 : Outport  Port=16
  wires:
  In1/1 -> ETMX/1(In1)
  In2/1 -> ETMX/2(In2)
  In3/1 -> ETMX/3(In3)
  In4/1 -> ETMX/4(In4)
  In5/1 -> ETMX/5(In5)
  In6/1 -> ETMX/6(In6)
  In7/1 -> ETMX/7(In7)
  In8/1 -> ETMX/8(In8)
  In9/1 -> ETMX/9(In9)
  In10/1 -> ETMX/10(In10)
  In11/1 -> ETMX/11(In11)
  In12/1 -> ETMX/12(In12)
  In13/1 -> ETMX/13(In13)
  In14/1 -> ETMX/14(In14)
  In15/1 -> ETMX/15(In15)
  In16/1 -> ETMX/16(In16)
  ETMX/1(Out1) -> Out1/1
  ETMX/2(Out2) -> Out2/1
  ETMX/3(Out3) -> Out3/1
  ETMX/4(Out4) -> Out4/1
  ETMX/5(Out5) -> Out5/1
  ETMX/6(Out6) -> Out6/1
  ETMX/7(Out7) -> Out7/1
  ETMX/8(Out8) -> Out8/1
  ETMX/9(Out9) -> Out9/1
  ETMX/10(Out10) -> Out10/1
  ETMX/11(Out11) -> Out11/1
  ETMX/12(Out12) -> Out12/1
  ETMX/13(Out13) -> Out13/1
  ETMX/14(Out14) -> Out14/1
  ETMX/15(Out15) -> Out15/1
  ETMX/16(Out16) -> Out16/1

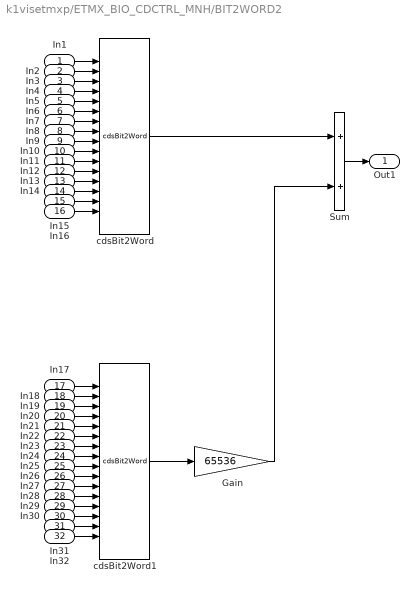
== system k1visetmxp/ETMX_BIO_CDCTRL_MNH/BIT2WORD2 ==
  In1 : Inport
  In2 : Inport  Port=2
  In3 : Inport  Port=3
  In4 : Inport  Port=4
  In5 : Inport  Port=5
  In6 : Inport  Port=6
  In7 : Inport  Port=7
  In8 : Inport  Port=8
  In9 : Inport  Port=9
  In10 : Inport  Port=10
  In11 : Inport  Port=11
  In12 : Inport  Port=12
  In13 : Inport  Port=13
  In14 : Inport  Port=14
  In15 : Inport  Port=15
  In16 : Inport  Port=16
  In17 : Inport  Port=17
  In18 : Inport  Port=18
  In19 : Inport  Port=19
  In20 : Inport  Port=20
  In21 : Inport  Port=21
  In22 : Inport  Port=22
  In23 : Inport  Port=23
  In24 : Inport  Port=24
  In25 : Inport  Port=25
  In26 : Inport  Port=26
  In27 : Inport  Port=27
  In28 : Inport  Port=28
  In29 : Inport  Port=29
  In30 : Inport  Port=30
  In31 : Inport  Port=31
  In32 : Inport  Port=32
  Gain : Gain  Gain=65536
  Sum : Sum
  cdsBit2Word : cdsBit2Word/cdsBit2Word  Tag=cdsBit2Word  Description=Forms single 16 bit integer from 16 0/1 inputs.
      settings: AttributesFormatString=%<Tag>
  cdsBit2Word1 : cdsBit2Word/cdsBit2Word  Tag=cdsBit2Word  Description=Forms single 16 bit integer from 16 0/1 inputs.
      settings: AttributesFormatString=%<Tag>
  Out1 : Outport
  wires:
  In32/1 -> cdsBit2Word1/16
  In31/1 -> cdsBit2Word1/15
  In30/1 -> cdsBit2Word1/14
  In29/1 -> cdsBit2Word1/13
  In28/1 -> cdsBit2Word1/12
  In27/1 -> cdsBit2Word1/11
  In26/1 -> cdsBit2Word1/10
  In25/1 -> cdsBit2Word1/9
  In24/1 -> cdsBit2Word1/8
  In23/1 -> cdsBit2Word1/7
  In22/1 -> cdsBit2Word1/6
  In21/1 -> cdsBit2Word1/5
  In20/1 -> cdsBit2Word1/4
  In19/1 -> cdsBit2Word1/3
  In18/1 -> cdsBit2Word1/2
  In17/1 -> cdsBit2Word1/1
  In16/1 -> cdsBit2Word/16
  In15/1 -> cdsBit2Word/15
  In14/1 -> cdsBit2Word/14
  In13/1 -> cdsBit2Word/13
  In12/1 -> cdsBit2Word/12
  In11/1 -> cdsBit2Word/11
  Sum/1 -> Out1/1
  In10/1 -> cdsBit2Word/10
  In9/1 -> cdsBit2Word/9
  In8/1 -> cdsBit2Word/8
  In7/1 -> cdsBit2Word/7
  In6/1 -> cdsBit2Word/6
  In5/1 -> cdsBit2Word/5
  In4/1 -> cdsBit2Word/4
  In3/1 -> cdsBit2Word/3
  In2/1 -> cdsBit2Word/2
  In1/1 -> cdsBit2Word/1
  cdsBit2Word/1 -> Sum/1
  cdsBit2Word1/1 -> Gain/1
  Gain/1 -> Sum/2

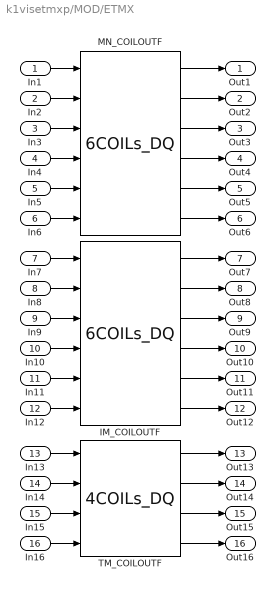
== system k1visetmxp/MOD/ETMX ==
  In1 : Inport
  In2 : Inport  Port=2
  In3 : Inport  Port=3
  In4 : Inport  Port=4
  In5 : Inport  Port=5
  In6 : Inport  Port=6
  In7 : Inport  Port=7
  In8 : Inport  Port=8
  In9 : Inport  Port=9
  In10 : Inport  Port=10
  In11 : Inport  Port=11
  In12 : Inport  Port=12
  In13 : Inport  Port=13
  In14 : Inport  Port=14
  In15 : Inport  Port=15
  In16 : Inport  Port=16
  IM_COILOUTF : VIS_LIB/UTILs/6COILs_DQ
  MN_COILOUTF : VIS_LIB/UTILs/6COILs_DQ
  TM_COILOUTF : VIS_LIB/UTILs/4COILs_DQ
  Out1 : Outport
  Out2 : Outport  Port=2
  Out3 : Outport  Port=3
  Out4 : Outport  Port=4
  Out5 : Outport  Port=5
  Out6 : Outport  Port=6
  Out7 : Outport  Port=7
  Out8 : Outport  Port=8
  Out9 : Outport  Port=9
  Out10 : Outport  Port=10
  Out11 : Outport  Port=11
  Out12 : Outport  Port=12
  Out13 : Outport  Port=13
  Out14 : Outport  Port=14
  Out15 : Outport  Port=15
  Out16 : Outport  Port=16
  wires:
  In4/1 -> MN_COILOUTF/4
  MN_COILOUTF/1 -> Out1/1
  In16/1 -> TM_COILOUTF/4
  TM_COILOUTF/1 -> Out13/1
  TM_COILOUTF/3 -> Out15/1
  In13/1 -> TM_COILOUTF/1
  In14/1 -> TM_COILOUTF/2
  In15/1 -> TM_COILOUTF/3
  TM_COILOUTF/2 -> Out14/1
  TM_COILOUTF/4 -> Out16/1
  In10/1 -> IM_COILOUTF/4
  IM_COILOUTF/1 -> Out7/1
  IM_COILOUTF/3 -> Out9/1
  In11/1 -> IM_COILOUTF/5
  In7/1 -> IM_COILOUTF/1
  In8/1 -> IM_COILOUTF/2
  In9/1 -> IM_COILOUTF/3
  IM_COILOUTF/5 -> Out11/1
  IM_COILOUTF/6 -> Out12/1
  In12/1 -> IM_COILOUTF/6
  IM_COILOUTF/2 -> Out8/1
  IM_COILOUTF/4 -> Out10/1
  MN_COILOUTF/3 -> Out3/1
  In5/1 -> MN_COILOUTF/5
  In1/1 -> MN_COILOUTF/1
  In2/1 -> MN_COILOUTF/2
  MN_COILOUTF/5 -> Out5/1
  In3/1 -> MN_COILOUTF/3
  In6/1 -> MN_COILOUTF/6
  MN_COILOUTF/6 -> Out6/1
  MN_COILOUTF/2 -> Out2/1
  MN_COILOUTF/4 -> Out4/1
